simulink model "slb_enb_reset"  (R2015b)
settings: Solver=FixedStepDiscrete  SolverMode=SingleTasking  StartTime=0.0  StopTime=20  RelTol=1e-3
StopFcn:
  | % my_logic
libraries: simulink x6
settings Model: Creator=at-mt  LastModifiedBy=amatsumo
settings DataIOCC: SaveFormat=Array  SignalLoggingSaveFormat=ModelDataLogs  SaveOutput=off  SignalLogging=off  SaveTime=off
settings OptimizationCC: BlockReduction=off  ConditionallyExecuteInputs=off  DefaultParameterBehavior=Inlined  ExpressionDepthLimit=2147483647
settings DebuggingCC: AlgebraicLoopMsg=error  UnderspecifiedInitializationDetection=Classic  MergeDetectMultiDrivingBlocksExec=none  SolverPrmCheckMsg=warning  SingleTaskRateTransMsg=error  FcnCallInpInsideContextMsg=UseLocalSettings  StateNameClashWarn=warning
settings HardwareCC: ProdBitPerPointer=32  ProdLargestAtomicFloat=None  ProdIntDivRoundTo=Undefined  ProdEndianess=Unspecified  ProdWordSize=32  ProdHWDeviceType=ASIC/FPGA->ASIC/FPGA  ProdEqTarget=off
settings GRTTargetCC: GeneratePreprocessorConditionals=Disable all  CombineOutputUpdateFcns=off  GRTInterface=on
settings ConfigComp: CovModelRefEnable=Off  CovSFcnEnable=off

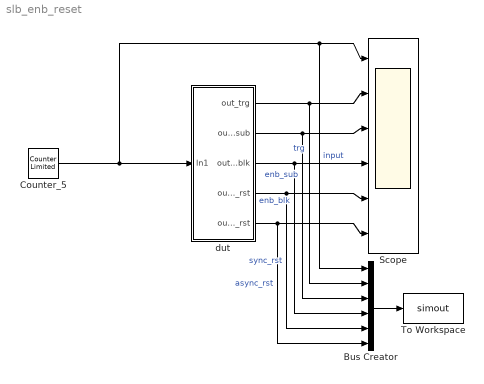
== system slb_enb_reset ==
  Bus Creator : BusCreator  Inputs=6
  Counter_5 : simulink/Sources/Counter Limited  uplimit=8  tsamp=1
  Scope : Scope  NumInputPorts=6
  To Workspace : ToWorkspace  VariableName=simout  SaveFormat=Timeseries  SampleTime=-1
  dut : Subsystem
  wires:
  Counter_5/1 -> Bus Creator/1, Scope/1, dut/1(In1)  "input"
  Bus Creator/1 -> To Workspace/1
  dut/3(out_enbblk) -> Bus Creator/4, Scope/4  "enb_blk"
  dut/4(out_sync_rst) -> Bus Creator/5, Scope/5  "sync_rst"
  dut/2(out_enbsub) -> Bus Creator/3, Scope/3  "enb_sub"
  dut/5(out_async_rst) -> Bus Creator/6, Scope/6  "async_rst"
  dut/1(out_trg) -> Bus Creator/2, Scope/2  "trg"

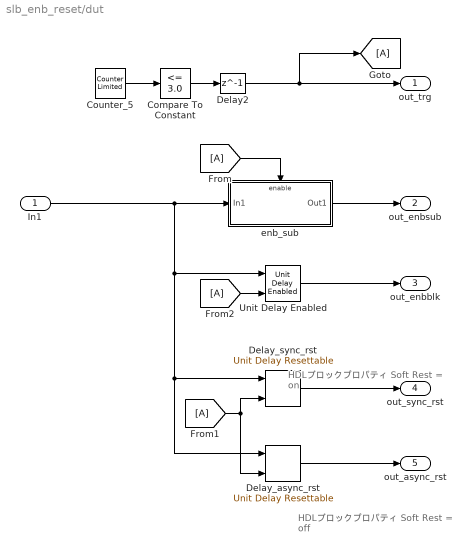
== system slb_enb_reset/dut ==
  note: HDLブロックプロパティ Soft Rest = off
  note: HDLブロックプロパティ Soft Rest = on
  In1 : Inport
  " Delay_async_rst" : simulink/Additional Math & Discrete/Additional Discrete/Unit Delay Resettable  vinit=0.0  tsamp=-1
  " Delay_sync_rst" : simulink/Additional Math & Discrete/Additional Discrete/Unit Delay Resettable  vinit=0.0  tsamp=-1
  Compare To Constant : simulink/Logic and Bit Operations/Compare To Constant  relop=<=  const=3.0  OutDataTypeStr=boolean
  Counter_5 : simulink/Sources/Counter Limited  uplimit=6  tsamp=1
  Delay2 : Delay  DelayLength=1  InputProcessing=Inherited
  Unit Delay Enabled : simulink/Additional Math & Discrete/Additional Discrete/Unit Delay Enabled  vinit=0.0  tsamp=-1
  enb_sub : Subsystem  TreatAsAtomicUnit=on
  out_trg : Outport
  out_enbsub : Outport  Port=2
  out_enbblk : Outport  Port=3
  out_sync_rst : Outport  Port=4
  out_async_rst : Outport  Port=5
  wires:
  In1/1 -> Unit Delay Enabled/1, " Delay_async_rst"/1, " Delay_sync_rst"/1, enb_sub/1(In1)
  Counter_5/1 -> Compare To Constant/1
  Compare To Constant/1 -> Delay2/1
  Delay2/1 -> [A], out_trg/1
  enb_sub/1(Out1) -> out_enbsub/1
  " Delay_sync_rst"/1 -> out_sync_rst/1
  " Delay_async_rst"/1 -> out_async_rst/1
  [A] -> enb_sub/Enable
  [A] -> " Delay_async_rst"/2, " Delay_sync_rst"/2
  [A] -> Unit Delay Enabled/2
  Unit Delay Enabled/1 -> out_enbblk/1

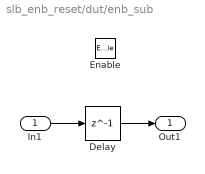
== system slb_enb_reset/dut/enb_sub ==
  In1 : Inport
  Enable : EnablePort
  Delay : Delay  DelayLength=1
  Out1 : Outport  InitialOutput=0
  wires:
  In1/1 -> Delay/1
  Delay/1 -> Out1/1
